simulink model "Normal_Multiplier"  (R2021a)
settings: Solver=FixedStepAuto  StartTime=0.0  StopTime=322.56  FixedStep=0.01  RelTol=1e-3
(part 3 of 3)

== system Normal_Multiplier/Full Adder52/Half Adder ==
  In : Inport
  Cin : Inport  Port=2
  Logical Operator : Logic  Operator=XOR  AllPortsSameDT=off  OutDataTypeStr=boolean
  Logical Operator1 : Logic  AllPortsSameDT=off  OutDataTypeStr=boolean
  Sum : Outport
  Cout : Outport  Port=2
  wires:
  In/1 -> Logical Operator1/1, Logical Operator/1
  Cin/1 -> Logical Operator/2, Logical Operator1/2
  Logical Operator/1 -> Sum/1
  Logical Operator1/1 -> Cout/1

== system Normal_Multiplier/Full Adder52/Half Adder1 ==
  In : Inport
  Cin : Inport  Port=2
  Logical Operator : Logic  Operator=XOR  AllPortsSameDT=off  OutDataTypeStr=boolean
  Logical Operator1 : Logic  AllPortsSameDT=off  OutDataTypeStr=boolean
  Sum : Outport
  Cout : Outport  Port=2
  wires:
  In/1 -> Logical Operator1/1, Logical Operator/1
  Cin/1 -> Logical Operator/2, Logical Operator1/2
  Logical Operator/1 -> Sum/1
  Logical Operator1/1 -> Cout/1

== system Normal_Multiplier/Full Adder53/Half Adder ==
  In : Inport
  Cin : Inport  Port=2
  Logical Operator : Logic  Operator=XOR  AllPortsSameDT=off  OutDataTypeStr=boolean
  Logical Operator1 : Logic  AllPortsSameDT=off  OutDataTypeStr=boolean
  Sum : Outport
  Cout : Outport  Port=2
  wires:
  In/1 -> Logical Operator1/1, Logical Operator/1
  Cin/1 -> Logical Operator/2, Logical Operator1/2
  Logical Operator/1 -> Sum/1
  Logical Operator1/1 -> Cout/1

== system Normal_Multiplier/Full Adder53/Half Adder1 ==
  In : Inport
  Cin : Inport  Port=2
  Logical Operator : Logic  Operator=XOR  AllPortsSameDT=off  OutDataTypeStr=boolean
  Logical Operator1 : Logic  AllPortsSameDT=off  OutDataTypeStr=boolean
  Sum : Outport
  Cout : Outport  Port=2
  wires:
  In/1 -> Logical Operator1/1, Logical Operator/1
  Cin/1 -> Logical Operator/2, Logical Operator1/2
  Logical Operator/1 -> Sum/1
  Logical Operator1/1 -> Cout/1

== system Normal_Multiplier/Full Adder55/Half Adder ==
  In : Inport
  Cin : Inport  Port=2
  Logical Operator : Logic  Operator=XOR  AllPortsSameDT=off  OutDataTypeStr=boolean
  Logical Operator1 : Logic  AllPortsSameDT=off  OutDataTypeStr=boolean
  Sum : Outport
  Cout : Outport  Port=2
  wires:
  In/1 -> Logical Operator1/1, Logical Operator/1
  Cin/1 -> Logical Operator/2, Logical Operator1/2
  Logical Operator/1 -> Sum/1
  Logical Operator1/1 -> Cout/1

== system Normal_Multiplier/Full Adder55/Half Adder1 ==
  In : Inport
  Cin : Inport  Port=2
  Logical Operator : Logic  Operator=XOR  AllPortsSameDT=off  OutDataTypeStr=boolean
  Logical Operator1 : Logic  AllPortsSameDT=off  OutDataTypeStr=boolean
  Sum : Outport
  Cout : Outport  Port=2
  wires:
  In/1 -> Logical Operator1/1, Logical Operator/1
  Cin/1 -> Logical Operator/2, Logical Operator1/2
  Logical Operator/1 -> Sum/1
  Logical Operator1/1 -> Cout/1

== system Normal_Multiplier/Full Adder56/Half Adder ==
  In : Inport
  Cin : Inport  Port=2
  Logical Operator : Logic  Operator=XOR  AllPortsSameDT=off  OutDataTypeStr=boolean
  Logical Operator1 : Logic  AllPortsSameDT=off  OutDataTypeStr=boolean
  Sum : Outport
  Cout : Outport  Port=2
  wires:
  In/1 -> Logical Operator1/1, Logical Operator/1
  Cin/1 -> Logical Operator/2, Logical Operator1/2
  Logical Operator/1 -> Sum/1
  Logical Operator1/1 -> Cout/1

== system Normal_Multiplier/Full Adder56/Half Adder1 ==
  In : Inport
  Cin : Inport  Port=2
  Logical Operator : Logic  Operator=XOR  AllPortsSameDT=off  OutDataTypeStr=boolean
  Logical Operator1 : Logic  AllPortsSameDT=off  OutDataTypeStr=boolean
  Sum : Outport
  Cout : Outport  Port=2
  wires:
  In/1 -> Logical Operator1/1, Logical Operator/1
  Cin/1 -> Logical Operator/2, Logical Operator1/2
  Logical Operator/1 -> Sum/1
  Logical Operator1/1 -> Cout/1

== system Normal_Multiplier/Full Adder6/Half Adder ==
  In : Inport
  Cin : Inport  Port=2
  Logical Operator : Logic  Operator=XOR  AllPortsSameDT=off  OutDataTypeStr=boolean
  Logical Operator1 : Logic  AllPortsSameDT=off  OutDataTypeStr=boolean
  Sum : Outport
  Cout : Outport  Port=2
  wires:
  In/1 -> Logical Operator1/1, Logical Operator/1
  Cin/1 -> Logical Operator/2, Logical Operator1/2
  Logical Operator/1 -> Sum/1
  Logical Operator1/1 -> Cout/1

== system Normal_Multiplier/Full Adder6/Half Adder1 ==
  In : Inport
  Cin : Inport  Port=2
  Logical Operator : Logic  Operator=XOR  AllPortsSameDT=off  OutDataTypeStr=boolean
  Logical Operator1 : Logic  AllPortsSameDT=off  OutDataTypeStr=boolean
  Sum : Outport
  Cout : Outport  Port=2
  wires:
  In/1 -> Logical Operator1/1, Logical Operator/1
  Cin/1 -> Logical Operator/2, Logical Operator1/2
  Logical Operator/1 -> Sum/1
  Logical Operator1/1 -> Cout/1

== system Normal_Multiplier/Full Adder8/Half Adder ==
  In : Inport
  Cin : Inport  Port=2
  Logical Operator : Logic  Operator=XOR  AllPortsSameDT=off  OutDataTypeStr=boolean
  Logical Operator1 : Logic  AllPortsSameDT=off  OutDataTypeStr=boolean
  Sum : Outport
  Cout : Outport  Port=2
  wires:
  In/1 -> Logical Operator1/1, Logical Operator/1
  Cin/1 -> Logical Operator/2, Logical Operator1/2
  Logical Operator/1 -> Sum/1
  Logical Operator1/1 -> Cout/1

== system Normal_Multiplier/Full Adder8/Half Adder1 ==
  In : Inport
  Cin : Inport  Port=2
  Logical Operator : Logic  Operator=XOR  AllPortsSameDT=off  OutDataTypeStr=boolean
  Logical Operator1 : Logic  AllPortsSameDT=off  OutDataTypeStr=boolean
  Sum : Outport
  Cout : Outport  Port=2
  wires:
  In/1 -> Logical Operator1/1, Logical Operator/1
  Cin/1 -> Logical Operator/2, Logical Operator1/2
  Logical Operator/1 -> Sum/1
  Logical Operator1/1 -> Cout/1

== system Normal_Multiplier/Full Adder9/Half Adder ==
  In : Inport
  Cin : Inport  Port=2
  Logical Operator : Logic  Operator=XOR  AllPortsSameDT=off  OutDataTypeStr=boolean
  Logical Operator1 : Logic  AllPortsSameDT=off  OutDataTypeStr=boolean
  Sum : Outport
  Cout : Outport  Port=2
  wires:
  In/1 -> Logical Operator1/1, Logical Operator/1
  Cin/1 -> Logical Operator/2, Logical Operator1/2
  Logical Operator/1 -> Sum/1
  Logical Operator1/1 -> Cout/1

== system Normal_Multiplier/Full Adder9/Half Adder1 ==
  In : Inport
  Cin : Inport  Port=2
  Logical Operator : Logic  Operator=XOR  AllPortsSameDT=off  OutDataTypeStr=boolean
  Logical Operator1 : Logic  AllPortsSameDT=off  OutDataTypeStr=boolean
  Sum : Outport
  Cout : Outport  Port=2
  wires:
  In/1 -> Logical Operator1/1, Logical Operator/1
  Cin/1 -> Logical Operator/2, Logical Operator1/2
  Logical Operator/1 -> Sum/1
  Logical Operator1/1 -> Cout/1
